simulink model "Nadir_Pointing"  (R2023b)
settings: Solver=VariableStepAuto  StartTime=0.0  StopTime=10.0  RelTol=1e-3
values from neighbouring files (symbols this model uses):
  a = 7259    [Group_51.m]
  a_sun = 149.60e6    (= 149600000)    [Group_51.m]
  ARW = (((arw*pi/180)/(sqrt(n_t)))^2)*n_t    [Group_51.m]
  Beta_CMG = acos(dot([1;0;0],uv_pyr))    [Group_51.m]
  delta_0_P = SM.delta_g_SM(end,:)    [Group_51.m]
  e = 0.001    [Group_51.m]
  e_sun = 0.0167086    [Group_51.m]
  eps_b = 11.5*pi/180    (= 0.200712863979)    [Group_51.m]
  eps_sun = deg2rad(23.45)    [Group_51.m]
  f0_P = SM.Theta_SM(end,1)    [Group_51.m]
  g_1_0 = -29404.8    [Group_51.m]
  g_1_1 = -1450.9    [Group_51.m]
  Gain_G = eye(3,3)    [Group_51.m]
  h_1_1 = 4653.5    [Group_51.m]
  h_r = [0.5;0.5;0.5;0.5]    [Group_51.m]
  halfrange = pi/40    (= 0.0785398163397)    [Group_51.m]
  i = deg2rad(97.27276)    [Group_51.m]
  I_tot = I+Ip_1_transp+Ip_2_transp    [Group_51.m]
  I_tot_inv = I_tot\eye(3,3)    [Group_51.m]
  IC312_P = [phi312_P;theta312_P;psi312_P]    [Group_51.m]
  jb = [0.1; 0.1;0.1]    [Group_51.m]
  k_cmg = -1    [Group_51.m]
  kdx_P = 2    [Group_51.m]
  kdy_P = 2.365    [Group_51.m]
  kdz_P = 2.1    [Group_51.m]
  kpx_SM = 0.129*0.5    (= 0.0645)    [Group_51.m]
  kpy_P = 1.4*0.5    (= 0.7)    [Group_51.m]
  kpz_P = 1*0.5    (= 0.5)    [Group_51.m]
  Miss_G = [teta_g_x;teta_g_y;teta_g_z]    [Group_51.m]
  n = sqrt(mu/ a^3)    [Group_51.m]
  n_sun = 2*pi/(365.26*24*3600)    (= 1.99096676796e-07)    [Group_51.m]
  n_t = samp_t    (= 1)    [Group_51.m]
  OM = deg2rad(90)    [Group_51.m]
  Re = astroConstants(23)    [Group_51.m]
  RRW = (((rrw*pi/180)/(sqrt(n_t)))^2)*n_t    [Group_51.m]
  samp_t = 1/samp_freq    (= 1)    [Group_51.m]
  t_sun_P = tf_D+tf_SM    (= 550)    [Group_51.m]
  w = deg2rad(0)    [Group_51.m]
  w0_P = [wx_P;wy_P;wz_P]    [Group_51.m]
  we = we/3600    (= 7.29159776389e-06)    [Group_51.m]
undefined symbols (not defined in the file or in its folder): DiscIntNeverNeededParam
libraries: matrix_library x15, vrlib x11, simulink x6, hdlsllib x2, dspswit3 x1
(part 2 of 2)

== system Nadir_Pointing/Kinematics/Subsystem/Subsystem4 ==
  angles313 : Inport
  Enable : EnablePort
  Subsystem1 : Subsystem
  Subsystem12 : Subsystem
  angles312 : Outport
  wires:
  Subsystem12/1(Out1) -> Subsystem1/1(matrix313)  "matrix313"
  Subsystem1/1(angles312) -> angles312/1  "angles312"
  angles313/1 -> Subsystem12/1(angles313)

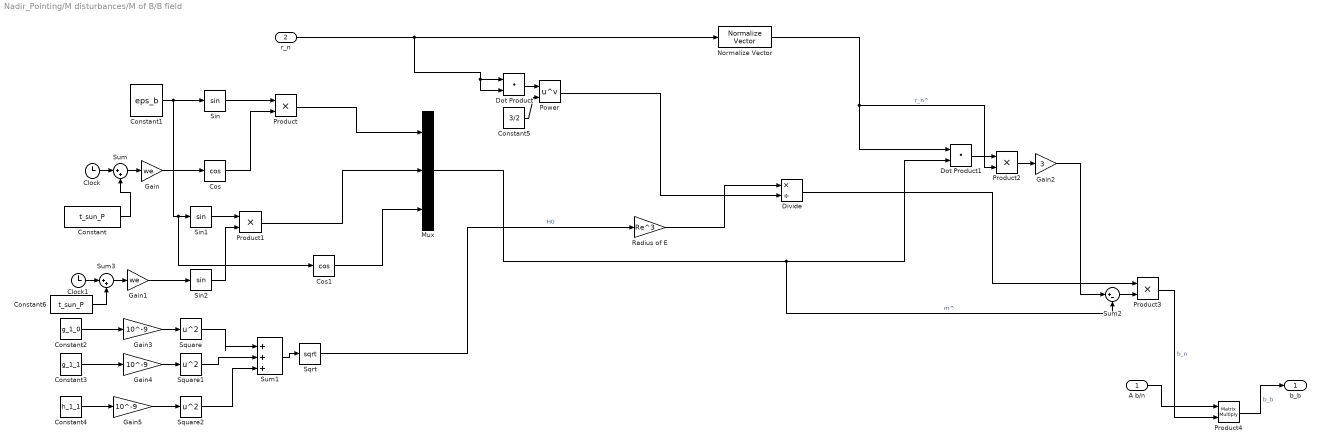
== system Nadir_Pointing/M disturbances/M of B/B field  ==
  A b/n : Inport
  r_n : Inport  Port=2
  Clock : Clock
  Clock1 : Clock
  Constant : Constant  Value=t_sun_P
  Constant1 : Constant  Value=eps_b
  Constant2 : Constant  Value=g_1_0
  Constant3 : Constant  Value=g_1_1
  Constant4 : Constant  Value=h_1_1
  Constant5 : Constant  Value=3/2
  Constant6 : Constant  Value=t_sun_P
  Cos : Trigonometry  Operator=cos
  Cos1 : Trigonometry  Operator=cos
  Divide : Product  Inputs=*/
  Dot Product : DotProduct  OutDataTypeStr=Inherit: Inherit via internal rule
  Dot Product1 : DotProduct  OutDataTypeStr=Inherit: Inherit via internal rule
  Gain : Gain  Gain=we
  Gain1 : Gain  Gain=we
  Gain2 : Gain  Gain=3
  Gain3 : Gain  Gain=10^-9
  Gain4 : Gain  Gain=10^-9
  Gain5 : Gain  Gain=10^-9
  Mux : Mux  Inputs=3
  Normalize Vector : vrlib/Utilities/Normalize Vector  maxzero=0
  Power : Math  Operator=pow
  Product{,1..3} (4 alike) : Product
  Product4 : Product  Multiplication=Matrix(*)
  Radius of E : Gain  Gain=Re^3
  Sin : Trigonometry
  Sin1 : Trigonometry
  Sin2 : Trigonometry
  Sqrt : Sqrt
  Square : Math  Operator=square
  Square1 : Math  Operator=square
  Square2 : Math  Operator=square
  Sum : Sum  Inputs=|++
  Sum1 : Sum  Inputs=|+++
  Sum2 : Sum  Inputs=|+-
  Sum3 : Sum  Inputs=|++
  b_b : Outport
  wires:
  A b/n/1 -> Product4/1
  Product2/1 -> Gain2/1
  Constant5/1 -> Power/2
  Radius of E/1 -> Divide/1
  Normalize Vector/1 -> Product2/2, Dot Product1/1  "r_n^"
  Gain/1 -> Cos/1
  Sum2/1 -> Product3/2
  Sin1/1 -> Product1/1
  Product1/1 -> Mux/2
  Sqrt/1 -> Radius of E/1  "H0"
  Gain1/1 -> Sin2/1
  Sin2/1 -> Product1/2
  Sin/1 -> Product/1
  Product4/1 -> b_b/1  "b_b"
  Cos/1 -> Product/2
  Square2/1 -> Sum1/3
  Constant1/1 -> Cos1/1, Sin1/1, Sin/1
  Cos1/1 -> Mux/3
  Dot Product/1 -> Power/1
  Product3/1 -> Product4/2  "b_n"
  Divide/1 -> Product3/1
  Product/1 -> Mux/1
  Power/1 -> Divide/2
  Sum1/1 -> Sqrt/1
  Dot Product1/1 -> Product2/1
  r_n/1 -> Normalize Vector/1, Dot Product/2, Dot Product/1
  Square1/1 -> Sum1/2
  Square/1 -> Sum1/1
  Mux/1 -> Sum2/2, Dot Product1/2  "m^"
  Gain2/1 -> Sum2/1
  Constant2/1 -> Gain3/1
  Gain3/1 -> Square/1
  Gain4/1 -> Square1/1
  Constant3/1 -> Gain4/1
  Constant4/1 -> Gain5/1
  Gain5/1 -> Square2/1
  Clock/1 -> Sum/1
  Sum/1 -> Gain/1
  Clock1/1 -> Sum3/1
  Sum3/1 -> Gain1/1
  Constant/1 -> Sum/2
  Constant6/1 -> Sum3/2

== system Nadir_Pointing/M disturbances/M of G G/D.C. of R  ==
  Ab/l : Inport
  Product : Product  Multiplication=Matrix(*)
  Yaw Axis : Constant  Value=[1; 0; 0]
  c : Outport
  wires:
  Product/1 -> c/1  "c"
  Ab/l/1 -> Product/1
  Yaw Axis/1 -> Product/2

== system Nadir_Pointing/Sensors/Gyroscopic Sensor/Skew ==
  Theta : Inport
  Constant1 : Constant  Value=[1;0;0]
  Constant2 : Constant  Value=[0;1;0]
  Constant3 : Constant  Value=[0;0;1]
  Cross Product : matrix_library/Cross Product
  Cross Product1 : matrix_library/Cross Product
  Cross Product2 : matrix_library/Cross Product
  Matrix Concatenate : Concatenate  NumInputs=3  Mode=Multidimensional array  ConcatenateDimension=2
  Skew_Theta : Outport
  wires:
  Cross Product/1 -> Matrix Concatenate/1
  Constant3/1 -> Cross Product2/2
  Constant1/1 -> Cross Product/2
  Cross Product1/1 -> Matrix Concatenate/2
  Matrix Concatenate/1 -> Skew_Theta/1
  Theta/1 -> Cross Product1/1, Cross Product2/1, Cross Product/1
  Cross Product2/1 -> Matrix Concatenate/3
  Constant2/1 -> Cross Product1/2

== system Nadir_Pointing/Control/Target Model/Subsystem1/2 A1 rot ==
  ang : Inport
  Constant1 : Constant  Value=[1 0 0; 0 0 0; 0 0 0]
  Constant2 : Constant  Value=[0 0 0; 0 1 0; 0 0 1]
  Constant3 : Constant  Value=[0 0 0; 0 0 1; 0 -1 0]
  Cos : Trigonometry  Operator=cos
  Product : Product
  Product1 : Product
  Sin : Trigonometry
  Sum : Sum  Inputs=|+||+||+
  A21 : Outport
  wires:
  ang/1 -> Sin/1, Cos/1
  Constant3/1 -> Product1/2
  Product1/1 -> Sum/3
  Product/1 -> Sum/2
  Constant1/1 -> Sum/1
  Sin/1 -> Product1/1
  Constant2/1 -> Product/2
  Cos/1 -> Product/1
  Sum/1 -> A21/1

== system Nadir_Pointing/Control/Target Model/Subsystem1/2 A3 rot ==
  ang : Inport
  Constant1 : Constant  Value=[0 0 0; 0 0 0; 0 0 1]
  Constant2 : Constant  Value=[1 0 0; 0 1 0; 0 0 0]
  Constant3 : Constant  Value=[0 1 0; -1 0 0; 0 0 0]
  Cos : Trigonometry  Operator=cos
  Product : Product
  Product1 : Product
  Sin : Trigonometry
  Sum : Sum  Inputs=|+||+||+
  A23 : Outport
  wires:
  Constant2/1 -> Product/2
  Sum/1 -> A23/1
  ang/1 -> Sin/1, Cos/1
  Product/1 -> Sum/2
  Cos/1 -> Product/1
  Sin/1 -> Product1/1
  Constant3/1 -> Product1/2
  Constant1/1 -> Sum/1
  Product1/1 -> Sum/3

== system Nadir_Pointing/Control/Target Model/Subsystem1/2 A3 rot2 ==
  ang : Inport
  Constant1 : Constant  Value=[0 0 0; 0 0 0; 0 0 1]
  Constant2 : Constant  Value=[1 0 0; 0 1 0; 0 0 0]
  Constant3 : Constant  Value=[0 1 0; -1 0 0; 0 0 0]
  Cos : Trigonometry  Operator=cos
  Product : Product
  Product1 : Product
  Sin : Trigonometry
  Sum : Sum  Inputs=|+||+||+
  A233 : Outport
  wires:
  Constant2/1 -> Product/2
  Sum/1 -> A233/1
  ang/1 -> Sin/1, Cos/1
  Product/1 -> Sum/2
  Cos/1 -> Product/1
  Sin/1 -> Product1/1
  Constant3/1 -> Product1/2
  Constant1/1 -> Sum/1
  Product1/1 -> Sum/3

== system Nadir_Pointing/Environment/A l//n for elliptical orbit/Subsystem1/2 A1 rot ==
  ang : Inport
  Constant1 : Constant  Value=[1 0 0; 0 0 0; 0 0 0]
  Constant2 : Constant  Value=[0 0 0; 0 1 0; 0 0 1]
  Constant3 : Constant  Value=[0 0 0; 0 0 1; 0 -1 0]
  Cos : Trigonometry  Operator=cos
  Product : Product
  Product1 : Product
  Sin : Trigonometry
  Sum : Sum  Inputs=|+||+||+
  A21 : Outport
  wires:
  ang/1 -> Sin/1, Cos/1
  Constant3/1 -> Product1/2
  Product1/1 -> Sum/3
  Product/1 -> Sum/2
  Constant1/1 -> Sum/1
  Sin/1 -> Product1/1
  Constant2/1 -> Product/2
  Cos/1 -> Product/1
  Sum/1 -> A21/1

== system Nadir_Pointing/Environment/A l//n for elliptical orbit/Subsystem1/2 A3 rot ==
  ang : Inport
  Constant1 : Constant  Value=[0 0 0; 0 0 0; 0 0 1]
  Constant2 : Constant  Value=[1 0 0; 0 1 0; 0 0 0]
  Constant3 : Constant  Value=[0 1 0; -1 0 0; 0 0 0]
  Cos : Trigonometry  Operator=cos
  Product : Product
  Product1 : Product
  Sin : Trigonometry
  Sum : Sum  Inputs=|+||+||+
  A23 : Outport
  wires:
  Constant2/1 -> Product/2
  Sum/1 -> A23/1
  ang/1 -> Sin/1, Cos/1
  Product/1 -> Sum/2
  Cos/1 -> Product/1
  Sin/1 -> Product1/1
  Constant3/1 -> Product1/2
  Constant1/1 -> Sum/1
  Product1/1 -> Sum/3

== system Nadir_Pointing/Environment/A l//n for elliptical orbit/Subsystem1/2 A3 rot2 ==
  ang : Inport
  Constant1 : Constant  Value=[0 0 0; 0 0 0; 0 0 1]
  Constant2 : Constant  Value=[1 0 0; 0 1 0; 0 0 0]
  Constant3 : Constant  Value=[0 1 0; -1 0 0; 0 0 0]
  Cos : Trigonometry  Operator=cos
  Product : Product
  Product1 : Product
  Sin : Trigonometry
  Sum : Sum  Inputs=|+||+||+
  A233 : Outport
  wires:
  Constant2/1 -> Product/2
  Sum/1 -> A233/1
  ang/1 -> Sin/1, Cos/1
  Product/1 -> Sum/2
  Cos/1 -> Product/1
  Sin/1 -> Product1/1
  Constant3/1 -> Product1/2
  Constant1/1 -> Sum/1
  Product1/1 -> Sum/3

== system Nadir_Pointing/Environment/Kep 2bp/Subsystem/2 A1 rot ==
  theta2 : Inport
  Constant1 : Constant  Value=[1 0 0; 0 0 0; 0 0 0]
  Constant2 : Constant  Value=[0 0 0; 0 1 0; 0 0 1]
  Constant3 : Constant  Value=[0 0 0; 0 0 1; 0 -1 0]
  Cos : Trigonometry  Operator=cos
  Product : Product
  Product1 : Product
  Sin : Trigonometry
  Sum : Sum  Inputs=|+||+||+
  A21 : Outport
  wires:
  theta2/1 -> Sin/1, Cos/1
  Constant3/1 -> Product1/2
  Product1/1 -> Sum/3
  Product/1 -> Sum/2
  Constant1/1 -> Sum/1
  Sin/1 -> Product1/1
  Constant2/1 -> Product/2
  Cos/1 -> Product/1
  Sum/1 -> A21/1

== system Nadir_Pointing/Environment/Kep 2bp/Subsystem/2 A3 rot ==
  angolo : Inport
  Constant1 : Constant  Value=[0 0 0; 0 0 0; 0 0 1]
  Constant2 : Constant  Value=[1 0 0; 0 1 0; 0 0 0]
  Constant3 : Constant  Value=[0 1 0; -1 0 0; 0 0 0]
  Cos : Trigonometry  Operator=cos
  Product : Product
  Product1 : Product
  Sin : Trigonometry
  Sum : Sum  Inputs=|+||+||+
  A23 : Outport
  wires:
  Constant2/1 -> Product/2
  Sum/1 -> A23/1
  angolo/1 -> Sin/1, Cos/1
  Product/1 -> Sum/2
  Cos/1 -> Product/1
  Sin/1 -> Product1/1
  Constant3/1 -> Product1/2
  Constant1/1 -> Sum/1
  Product1/1 -> Sum/3

== system Nadir_Pointing/Environment/Kep 2bp/Subsystem/2 A3 rot2 ==
  angolo : Inport
  Constant1 : Constant  Value=[0 0 0; 0 0 0; 0 0 1]
  Constant2 : Constant  Value=[1 0 0; 0 1 0; 0 0 0]
  Constant3 : Constant  Value=[0 1 0; -1 0 0; 0 0 0]
  Cos : Trigonometry  Operator=cos
  Product : Product
  Product1 : Product
  Sin : Trigonometry
  Sum : Sum  Inputs=|+||+||+
  A233 : Outport
  wires:
  Constant2/1 -> Product/2
  Sum/1 -> A233/1
  angolo/1 -> Sin/1, Cos/1
  Product/1 -> Sum/2
  Cos/1 -> Product/1
  Sin/1 -> Product1/1
  Constant3/1 -> Product1/2
  Constant1/1 -> Sum/1
  Product1/1 -> Sum/3

== system Nadir_Pointing/Kinematics/Euler Angles/Kinematics 312/Subsystem1 ==
  wx : Inport
  theta : Inport  Port=2
  wz : Inport  Port=3
  psi : Inport  Port=4
  Cos : Trigonometry  Operator=cos
  Cos1 : Trigonometry  Operator=cos
  Divide : Product  Inputs=*/
  Product : Product
  Product1 : Product
  Sin : Trigonometry
  Sum : Sum  Inputs=|+-
  Out1 : Outport
  wires:
  psi/1 -> Cos/1, Sin/1
  theta/1 -> Cos1/1
  Product1/1 -> Sum/2
  Sum/1 -> Divide/1
  Product/1 -> Sum/1
  Sin/1 -> Product1/1
  Cos1/1 -> Divide/2
  Cos/1 -> Product/2
  wx/1 -> Product1/2
  wz/1 -> Product/1
  Divide/1 -> Out1/1  "phidot"

== system Nadir_Pointing/Kinematics/Euler Angles/Kinematics 312/Subsystem3 ==
  wx : Inport
  wy : Inport  Port=2
  theta : Inport  Port=3
  psi : Inport  Port=4
  wz : Inport  Port=5
  Cos : Trigonometry  Operator=cos
  Cos1 : Trigonometry  Operator=cos
  Divide : Product  Inputs=*/
  Product : Product
  Product1 : Product
  Product2 : Product
  Sin : Trigonometry
  Sin1 : Trigonometry
  Subtract : Sum  Inputs=+-
  Subtract1 : Sum  Inputs=+-
  Out1 : Outport
  wires:
  psi/1 -> Cos/1, Sin/1
  Subtract/1 -> Product2/1
  Sin1/1 -> Divide/1
  Product2/1 -> Subtract1/2
  Sin/1 -> Product1/1
  Cos/1 -> Product/2
  Cos1/1 -> Divide/2
  Subtract1/1 -> Out1/1  "psidot"
  wz/1 -> Product/1
  theta/1 -> Sin1/1, Cos1/1
  Product1/1 -> Subtract/2
  Divide/1 -> Product2/2
  Product/1 -> Subtract/1
  wy/1 -> Subtract1/1
  wx/1 -> Product1/2

== system Nadir_Pointing/Kinematics/Euler Angles/Kinematics 312/Subsystem4 ==
  wx : Inport
  wz : Inport  Port=2
  psi : Inport  Port=3
  Cos : Trigonometry  Operator=cos
  Product : Product
  Product1 : Product
  Sin : Trigonometry
  Sum : Sum  Inputs=|++
  Out1 : Outport
  wires:
  Sum/1 -> Out1/1  "thetadot"
  Sin/1 -> Product1/1
  psi/1 -> Sin/1, Cos/1
  Product/1 -> Sum/1
  Product1/1 -> Sum/2
  wx/1 -> Product/1
  Cos/1 -> Product/2
  wz/1 -> Product1/2

== system Nadir_Pointing/Kinematics/Euler Angles/Kinematics 312/Subsystem5 ==
  psi312 : Inport
  Constant1 : Constant  Value=[0 0 0; 0 1 0; 0 0 0]
  Constant2 : Constant  Value=[0 0 -1; 0 0 0; 1 0 0]
  Constant3 : Constant  Value=[1 0 0; 0 0 0; 0 0 1]
  Cos : Trigonometry  Operator=cos
  Product : Product
  Product1 : Product
  Sin : Trigonometry
  Sum : Sum  Inputs=|+++
  2 : Outport
  wires:
  Sum/1 -> 2/1  "A2psi"
  psi312/1 -> Cos/1, Sin/1  "psi"
  Constant1/1 -> Sum/1
  Product/1 -> Sum/2
  Constant2/1 -> Product/2
  Sin/1 -> Product/1
  Cos/1 -> Product1/1
  Constant3/1 -> Product1/2
  Product1/1 -> Sum/3

== system Nadir_Pointing/Kinematics/Euler Angles/Kinematics 312/Subsystem7 ==
  theta312 : Inport
  Constant1 : Constant  Value=[1 0 0; 0 0 0; 0 0 0]
  Constant2 : Constant  Value=[0 0 0; 0 0 1; 0 -1 0]
  Constant3 : Constant  Value=[0 0 0; 0 1 0; 0 0 1]
  Cos : Trigonometry  Operator=cos
  Product : Product
  Product1 : Product
  Sin : Trigonometry
  Sum : Sum  Inputs=|+++
  1 : Outport
  wires:
  theta312/1 -> Cos/1, Sin/1
  Sum/1 -> 1/1  "A1theta"
  Constant1/1 -> Sum/1
  Sin/1 -> Product/1
  Constant2/1 -> Product/2
  Product/1 -> Sum/2
  Cos/1 -> Product1/1
  Constant3/1 -> Product1/2
  Product1/1 -> Sum/3

== system Nadir_Pointing/Kinematics/Euler Angles/Kinematics 312/Subsystem9 ==
  phi312 : Inport
  Constant1 : Constant  Value=[0 0 0; 0 0 0; 0 0 1]
  Constant2 : Constant  Value=[0 1 0; -1 0 0; 0 0 0]
  Constant3 : Constant  Value=[1 0 0; 0 1 0; 0 0 0]
  Cos : Trigonometry  Operator=cos
  Product : Product
  Product1 : Product
  Sin : Trigonometry
  Sum : Sum  Inputs=|+++
  3 : Outport
  wires:
  phi312/1 -> Cos/1, Sin/1
  Constant1/1 -> Sum/1
  Sum/1 -> 3/1  "A3phi"
  Sin/1 -> Product/1
  Constant2/1 -> Product/2
  Product/1 -> Sum/2
  Cos/1 -> Product1/1
  Constant3/1 -> Product1/2
  Product1/1 -> Sum/3

== system Nadir_Pointing/Kinematics/Euler Angles/Kinematics 313/Subsystem1 ==
  wx : Inport
  wy : Inport  Port=2
  psi : Inport  Port=3
  Cos : Trigonometry  Operator=cos
  Product : Product
  Product1 : Product
  Sin : Trigonometry
  Subtract : Sum  Inputs=-+
  thetadot : Outport
  wires:
  Product/1 -> Subtract/1
  Product1/1 -> Subtract/2
  psi/1 -> Sin/1, Cos/1
  wy/1 -> Product/1
  wx/1 -> Product1/2
  Cos/1 -> Product1/1
  Subtract/1 -> thetadot/1  "thetadot"
  Sin/1 -> Product/2

== system Nadir_Pointing/Kinematics/Euler Angles/Kinematics 313/Subsystem2 ==
  wx : Inport
  wy : Inport  Port=2
  theta : Inport  Port=3
  psi : Inport  Port=4
  Cos : Trigonometry  Operator=cos
  Cos1 : Trigonometry
  Divide : Product  Inputs=*/
  Product : Product
  Product1 : Product
  Sin : Trigonometry
  Sum : Sum  Inputs=|++
  phidot : Outport
  wires:
  psi/1 -> Cos/1, Sin/1
  Cos/1 -> Product/1
  Sum/1 -> Divide/1
  Cos1/1 -> Divide/2
  Product/1 -> Sum/2
  Product1/1 -> Sum/1
  Sin/1 -> Product1/1
  wx/1 -> Product1/2
  wy/1 -> Product/2
  Divide/1 -> phidot/1  "phidot"
  theta/1 -> Cos1/1

== system Nadir_Pointing/Kinematics/Euler Angles/Kinematics 313/Subsystem3 ==
  wx : Inport
  wy : Inport  Port=2
  theta : Inport  Port=3
  wz : Inport  Port=4
  psi : Inport  Port=5
  Cos : Trigonometry  Operator=cos
  Cos1 : Trigonometry
  Cos2 : Trigonometry  Operator=cos
  Cos3 : Trigonometry
  Divide : Product  Inputs=*/
  Product : Product
  Product1 : Product
  Product2 : Product
  Sum : Sum  Inputs=|++
  Sum1 : Sum  Inputs=+-
  psidot : Outport
  wires:
  theta/1 -> Cos3/1, Cos2/1
  Product2/1 -> Sum1/2
  Cos/1 -> Product1/1
  Product/1 -> Sum/1
  Cos2/1 -> Divide/1
  psi/1 -> Cos/1, Cos1/1
  Cos3/1 -> Divide/2
  Divide/1 -> Product2/2
  Sum/1 -> Product2/1
  wy/1 -> Product1/2
  Product1/1 -> Sum/2
  Sum1/1 -> psidot/1  "psidot"
  wz/1 -> Sum1/1
  Cos1/1 -> Product/2
  wx/1 -> Product/1

== system Nadir_Pointing/Kinematics/Euler Angles/Kinematics 313/Subsystem4 ==
  theta : Inport
  Constant1 : Constant  Value=[1 0 0; 0 0 0; 0 0 0]
  Constant2 : Constant  Value=[0 0 0; 0 0 1; 0 -1 0]
  Constant3 : Constant  Value=[0 0 0; 0 1 0; 0 0 1]
  Cos : Trigonometry  Operator=cos
  Product : Product
  Product1 : Product
  Sin : Trigonometry
  Sum : Sum  Inputs=|+++
  1 : Outport
  wires:
  theta/1 -> Cos/1, Sin/1
  Sum/1 -> 1/1  "A1theta"
  Constant1/1 -> Sum/1
  Sin/1 -> Product/1
  Constant2/1 -> Product/2
  Product/1 -> Sum/2
  Cos/1 -> Product1/1
  Constant3/1 -> Product1/2
  Product1/1 -> Sum/3

== system Nadir_Pointing/Kinematics/Euler Angles/Kinematics 313/Subsystem5 ==
  psi : Inport
  Constant1 : Constant  Value=[0 0 0; 0 0 0; 0 0 1]
  Constant2 : Constant  Value=[0 1 0; -1 0 0; 0 0 0]
  Constant3 : Constant  Value=[1 0 0; 0 1 0; 0 0 0]
  Cos : Trigonometry  Operator=cos
  Product : Product
  Product1 : Product
  Sin : Trigonometry
  Sum : Sum  Inputs=|+++
  3 : Outport
  wires:
  Sum/1 -> 3/1  "A3psi"
  psi/1 -> Sin/1, Cos/1  "psi"
  Product1/1 -> Sum/3
  Constant3/1 -> Product1/2
  Sin/1 -> Product/1
  Constant2/1 -> Product/2
  Cos/1 -> Product1/1
  Product/1 -> Sum/2
  Constant1/1 -> Sum/1

== system Nadir_Pointing/Kinematics/Euler Angles/Kinematics 313/Subsystem6 ==
  phi : Inport
  Constant1 : Constant  Value=[0 0 0; 0 0 0; 0 0 1]
  Constant2 : Constant  Value=[0 1 0; -1 0 0; 0 0 0]
  Constant3 : Constant  Value=[1 0 0; 0 1 0; 0 0 0]
  Cos : Trigonometry  Operator=cos
  Product : Product
  Product1 : Product
  Sin : Trigonometry
  Sum : Sum  Inputs=|+++
  3 : Outport
  wires:
  phi/1 -> Cos/1, Sin/1
  Constant1/1 -> Sum/1
  Sum/1 -> 3/1  "A3phi"
  Sin/1 -> Product/1
  Constant2/1 -> Product/2
  Product/1 -> Sum/2
  Cos/1 -> Product1/1
  Constant3/1 -> Product1/2
  Product1/1 -> Sum/3

== system Nadir_Pointing/Kinematics/Euler Angles/Subsystem3/Subsystem10 ==
  In1 : Inport
  Atan2 : Trigonometry  Operator=atan2
  Atan5 : Trigonometry  Operator=atan2
  Atan6 : Trigonometry  Operator=atan2
  Divide1 : Product  Inputs=*/
  Gain3 : Gain  Gain=-1
  Mux2 : Mux  Inputs=3
  Selector12 : Selector  NumberOfDimensions=2  InputPortWidth=3  IndexOptions=Index vector (dialog),Index vector (dialog)  Indices=3,1  OutputSizes=1,1
  Selector13 : Selector  NumberOfDimensions=2  InputPortWidth=3  IndexOptions=Index vector (dialog),Index vector (dialog)  Indices=3,2  OutputSizes=1,1
  Selector14 : Selector  NumberOfDimensions=2  InputPortWidth=3  IndexOptions=Index vector (dialog),Index vector (dialog)  Indices=1,3  OutputSizes=1,1
  Selector15 : Selector  NumberOfDimensions=2  InputPortWidth=3  IndexOptions=Index vector (dialog),Index vector (dialog)  Indices=2,3  OutputSizes=1,1
  Selector5 : Selector  NumberOfDimensions=2  InputPortWidth=3  IndexOptions=Index vector (dialog),Index vector (dialog)  Indices=3,3  OutputSizes=1,1
  Square Root1 : Sqrt
  Square4 : Math  Operator=square
  Square5 : Math  Operator=square
  Sum2 : Sum  Inputs=|++
  Tan2 : Trigonometry  Operator=atan
  angles313 : Outport
  wires:
  Square Root1/1 -> Atan6/1
  In1/1 -> Selector15/1, Selector14/1, Selector13/1, Selector5/1, Selector12/1  "matrix312"
  Atan5/1 -> Mux2/3  "psicheck"
  Selector13/1 -> Atan2/2, Divide1/2, Square5/1  "a32"
  Selector14/1 -> Atan5/1  "a13"
  Square5/1 -> Sum2/2
  Selector5/1 -> Atan6/2  "a33"
  Gain3/1 -> Mux2/1  "phicheck"
  Selector12/1 -> Atan2/1, Divide1/1, Square4/1  "a31"
  Selector15/1 -> Atan5/2  "a23"
  Atan6/1 -> Mux2/2  "thetacheck"
  Sum2/1 -> Square Root1/1
  Square4/1 -> Sum2/1
  Mux2/1 -> angles313/1  "angles313"
  Divide1/1 -> Tan2/1
  Atan2/1 -> Gain3/1

== system Nadir_Pointing/Kinematics/Euler Angles/Subsystem3/Subsystem12 ==
  angles313 : Inport
  Demux5 : Demux  Outputs=3
  Matrix Multiply1 : Product  Inputs=3  Multiplication=Matrix(*)
  Subsystem4 : Subsystem
  Subsystem5 : Subsystem
  Subsystem6 : Subsystem
  Out1 : Outport
  wires:
  Demux5/1 -> Subsystem6/1(phi)
  Subsystem4/1(1) -> Matrix Multiply1/2
  Subsystem6/1(3) -> Matrix Multiply1/3
  angles313/1 -> Demux5/1
  Subsystem5/1(3) -> Matrix Multiply1/1
  Demux5/3 -> Subsystem5/1(psi)
  Demux5/2 -> Subsystem4/1(theta)
  Matrix Multiply1/1 -> Out1/1  "matrix313"

== system Nadir_Pointing/Kinematics/Euler Angles/Subsystem3/Subsystem4 ==
  matrix313 : Inport
  Atan1 : Trigonometry  Operator=atan2
  Atan2 : Trigonometry  Operator=atan2
  Atan3 : Trigonometry  Operator=atan2
  Divide : Product  Inputs=*/
  Gain : Gain  Gain=-1
  Mux : Mux  Inputs=3
  Selector : Selector  NumberOfDimensions=2  InputPortWidth=3  IndexOptions=Index vector (dialog),Index vector (dialog)  Indices=3,3  OutputSizes=1,1
  Selector1 : Selector  NumberOfDimensions=2  InputPortWidth=3  IndexOptions=Index vector (dialog),Index vector (dialog)  Indices=3,1  OutputSizes=1,1
  Selector2 : Selector  NumberOfDimensions=2  InputPortWidth=3  IndexOptions=Index vector (dialog),Index vector (dialog)  Indices=3,2  OutputSizes=1,1
  Selector3 : Selector  NumberOfDimensions=2  InputPortWidth=3  IndexOptions=Index vector (dialog),Index vector (dialog)  Indices=1,3  OutputSizes=1,1
  Selector4 : Selector  NumberOfDimensions=2  InputPortWidth=3  IndexOptions=Index vector (dialog),Index vector (dialog)  Indices=2,3  OutputSizes=1,1
  Square : Math  Operator=square
  Square Root : Sqrt
  Square1 : Math  Operator=square
  Sum : Sum  Inputs=|++
  Tan : Trigonometry  Operator=atan
  angles313 : Outport
  wires:
  Atan1/1 -> Mux/3  "psicheck"
  Selector/1 -> Atan2/2  "a33"
  Square Root/1 -> Atan2/1
  Square1/1 -> Sum/2
  Square/1 -> Sum/1
  Selector4/1 -> Atan1/2  "a23"
  Sum/1 -> Square Root/1
  matrix313/1 -> Selector/1, Selector2/1, Selector3/1, Selector4/1, Selector1/1
  Gain/1 -> Mux/1  "phicheck"
  Selector3/1 -> Atan1/1  "a13"
  Selector2/1 -> Atan3/2, Divide/2, Square1/1  "a32"
  Divide/1 -> Tan/1
  Selector1/1 -> Atan3/1, Divide/1, Square/1  "a31"
  Atan2/1 -> Mux/2  "thetacheck"
  Mux/1 -> angles313/1  "angles313"
  Atan3/1 -> Gain/1

== system Nadir_Pointing/Kinematics/Euler Angles/Subsystem3/Subsystem6 ==
  In1 : Inport
  Demux : Demux  Outputs=3
  Matrix Multiply : Product  Inputs=3  Multiplication=Matrix(*)
  Subsystem7 : Subsystem
  Subsystem8 : Subsystem
  Subsystem9 : Subsystem
  Out1 : Outport
  wires:
  Subsystem7/1(2) -> Matrix Multiply/1
  Demux/1 -> Subsystem9/1(phi312)
  Demux/3 -> Subsystem7/1(psi312)
  Demux/2 -> Subsystem8/1(theta312)
  Subsystem8/1(1) -> Matrix Multiply/2
  Subsystem9/1(3) -> Matrix Multiply/3
  In1/1 -> Demux/1
  Matrix Multiply/1 -> Out1/1  "matrix312"

== system Nadir_Pointing/Kinematics/Euler Angles/Subsystem4/Subsystem1 ==
  matrix313 : Inport
  Atan3 : Trigonometry  Operator=atan2
  Atan4 : Trigonometry  Operator=atan2
  Display2 : Display
  Gain1 : Gain  Gain=-1
  Gain2 : Gain  Gain=-1
  Mux1 : Mux  Inputs=3
  Selector10 : Selector  NumberOfDimensions=2  InputPortWidth=3  IndexOptions=Index vector (dialog),Index vector (dialog)  Indices=1,3  OutputSizes=1,1
  Selector11 : Selector  NumberOfDimensions=2  InputPortWidth=3  IndexOptions=Index vector (dialog),Index vector (dialog)  Indices=3,3  OutputSizes=1,1
  Selector6 : Selector  NumberOfDimensions=2  InputPortWidth=3  IndexOptions=Index vector (dialog),Index vector (dialog)  Indices=3,3  OutputSizes=1,1
  Selector7 : Selector  NumberOfDimensions=2  InputPortWidth=3  IndexOptions=Index vector (dialog),Index vector (dialog)  Indices=2,3  OutputSizes=1,1
  Selector8 : Selector  NumberOfDimensions=2  InputPortWidth=3  IndexOptions=Index vector (dialog),Index vector (dialog)  Indices=2,1  OutputSizes=1,1
  Selector9 : Selector  NumberOfDimensions=2  InputPortWidth=3  IndexOptions=Index vector (dialog),Index vector (dialog)  Indices=2,2  OutputSizes=1,1
  Sqrt : Sqrt
  Square2 : Math  Operator=square
  Square3 : Math  Operator=square
  Sum1 : Sum  Inputs=|++
  Tan1 : Trigonometry  Operator=atan2
  angles312 : Outport
  wires:
  Selector9/1 -> Square3/1, Tan1/2  "a22"
  Sqrt/1 -> Atan3/2
  matrix313/1 -> Selector7/1, Selector8/1, Selector9/1, Selector11/1, Selector10/1, Selector6/1
  Selector8/1 -> Tan1/1, Square2/1  "a21"
  Selector10/1 -> Atan4/1  "a13"
  Gain2/1 -> Mux1/3  "psicheck"
  Square2/1 -> Sum1/1
  Sum1/1 -> Sqrt/1
  Selector11/1 -> Atan4/2  "a33"
  Selector6/1 -> Display2/1
  Square3/1 -> Sum1/2
  Selector7/1 -> Atan3/1  "a23"
  Atan4/1 -> Gain2/1
  Tan1/1 -> Gain1/1
  Atan3/1 -> Mux1/2  "thetacheck"
  Gain1/1 -> Mux1/1  "phicheck"
  Mux1/1 -> angles312/1  "angles312"

== system Nadir_Pointing/Kinematics/Euler Angles/Subsystem4/Subsystem12 ==
  angles313 : Inport
  Demux5 : Demux  Outputs=3
  Matrix Multiply1 : Product  Inputs=3  Multiplication=Matrix(*)
  Subsystem4 : Subsystem
  Subsystem5 : Subsystem
  Subsystem6 : Subsystem
  Out1 : Outport
  wires:
  Demux5/1 -> Subsystem6/1(phi)
  Subsystem4/1(1) -> Matrix Multiply1/2
  Subsystem6/1(3) -> Matrix Multiply1/3
  angles313/1 -> Demux5/1
  Subsystem5/1(3) -> Matrix Multiply1/1
  Demux5/3 -> Subsystem5/1(psi)
  Demux5/2 -> Subsystem4/1(theta)
  Matrix Multiply1/1 -> Out1/1  "matrix313"

== system Nadir_Pointing/Kinematics/Subsystem/Subsystem4/Subsystem1 ==
  matrix313 : Inport
  Atan3 : Trigonometry  Operator=atan2
  Atan4 : Trigonometry  Operator=atan2
  Display2 : Display
  Gain1 : Gain  Gain=-1
  Gain2 : Gain  Gain=-1
  Mux1 : Mux  Inputs=3
  Selector10 : Selector  NumberOfDimensions=2  InputPortWidth=3  IndexOptions=Index vector (dialog),Index vector (dialog)  Indices=1,3  OutputSizes=1,1
  Selector11 : Selector  NumberOfDimensions=2  InputPortWidth=3  IndexOptions=Index vector (dialog),Index vector (dialog)  Indices=3,3  OutputSizes=1,1
  Selector6 : Selector  NumberOfDimensions=2  InputPortWidth=3  IndexOptions=Index vector (dialog),Index vector (dialog)  Indices=3,3  OutputSizes=1,1
  Selector7 : Selector  NumberOfDimensions=2  InputPortWidth=3  IndexOptions=Index vector (dialog),Index vector (dialog)  Indices=2,3  OutputSizes=1,1
  Selector8 : Selector  NumberOfDimensions=2  InputPortWidth=3  IndexOptions=Index vector (dialog),Index vector (dialog)  Indices=2,1  OutputSizes=1,1
  Selector9 : Selector  NumberOfDimensions=2  InputPortWidth=3  IndexOptions=Index vector (dialog),Index vector (dialog)  Indices=2,2  OutputSizes=1,1
  Sqrt : Sqrt
  Square2 : Math  Operator=square
  Square3 : Math  Operator=square
  Sum1 : Sum  Inputs=|++
  Tan1 : Trigonometry  Operator=atan2
  angles312 : Outport
  wires:
  Selector9/1 -> Square3/1, Tan1/2  "a22"
  Sqrt/1 -> Atan3/2
  matrix313/1 -> Selector7/1, Selector8/1, Selector9/1, Selector11/1, Selector10/1, Selector6/1
  Selector8/1 -> Tan1/1, Square2/1  "a21"
  Selector10/1 -> Atan4/1  "a13"
  Gain2/1 -> Mux1/3  "psicheck"
  Square2/1 -> Sum1/1
  Sum1/1 -> Sqrt/1
  Selector11/1 -> Atan4/2  "a33"
  Selector6/1 -> Display2/1
  Square3/1 -> Sum1/2
  Selector7/1 -> Atan3/1  "a23"
  Atan4/1 -> Gain2/1
  Tan1/1 -> Gain1/1
  Atan3/1 -> Mux1/2  "thetacheck"
  Gain1/1 -> Mux1/1  "phicheck"
  Mux1/1 -> angles312/1  "angles312"

== system Nadir_Pointing/Kinematics/Subsystem/Subsystem4/Subsystem12 ==
  angles313 : Inport
  Demux5 : Demux  Outputs=3
  Matrix Multiply1 : Product  Inputs=3  Multiplication=Matrix(*)
  Subsystem4 : Subsystem
  Subsystem5 : Subsystem
  Subsystem6 : Subsystem
  Out1 : Outport
  wires:
  Demux5/1 -> Subsystem6/1(phi)
  Subsystem4/1(1) -> Matrix Multiply1/2
  Subsystem6/1(3) -> Matrix Multiply1/3
  angles313/1 -> Demux5/1
  Subsystem5/1(3) -> Matrix Multiply1/1
  Demux5/3 -> Subsystem5/1(psi)
  Demux5/2 -> Subsystem4/1(theta)
  Matrix Multiply1/1 -> Out1/1  "matrix313"

== system Nadir_Pointing/Kinematics/Euler Angles/Subsystem3/Subsystem12/Subsystem4 ==
  theta : Inport
  Constant1 : Constant  Value=[1 0 0; 0 0 0; 0 0 0]
  Constant2 : Constant  Value=[0 0 0; 0 0 1; 0 -1 0]
  Constant3 : Constant  Value=[0 0 0; 0 1 0; 0 0 1]
  Cos : Trigonometry  Operator=cos
  Product : Product
  Product1 : Product
  Sin : Trigonometry
  Sum : Sum  Inputs=|+++
  1 : Outport
  wires:
  theta/1 -> Cos/1, Sin/1
  Sum/1 -> 1/1  "A1theta"
  Constant1/1 -> Sum/1
  Sin/1 -> Product/1
  Constant2/1 -> Product/2
  Product/1 -> Sum/2
  Cos/1 -> Product1/1
  Constant3/1 -> Product1/2
  Product1/1 -> Sum/3

== system Nadir_Pointing/Kinematics/Euler Angles/Subsystem3/Subsystem12/Subsystem5 ==
  psi : Inport
  Constant1 : Constant  Value=[0 0 0; 0 0 0; 0 0 1]
  Constant2 : Constant  Value=[0 1 0; -1 0 0; 0 0 0]
  Constant3 : Constant  Value=[1 0 0; 0 1 0; 0 0 0]
  Cos : Trigonometry  Operator=cos
  Product : Product
  Product1 : Product
  Sin : Trigonometry
  Sum : Sum  Inputs=|+++
  3 : Outport
  wires:
  Sum/1 -> 3/1  "A3psi"
  psi/1 -> Sin/1, Cos/1  "psi"
  Product1/1 -> Sum/3
  Constant3/1 -> Product1/2
  Sin/1 -> Product/1
  Constant2/1 -> Product/2
  Cos/1 -> Product1/1
  Product/1 -> Sum/2
  Constant1/1 -> Sum/1

== system Nadir_Pointing/Kinematics/Euler Angles/Subsystem3/Subsystem12/Subsystem6 ==
  phi : Inport
  Constant1 : Constant  Value=[0 0 0; 0 0 0; 0 0 1]
  Constant2 : Constant  Value=[0 1 0; -1 0 0; 0 0 0]
  Constant3 : Constant  Value=[1 0 0; 0 1 0; 0 0 0]
  Cos : Trigonometry  Operator=cos
  Product : Product
  Product1 : Product
  Sin : Trigonometry
  Sum : Sum  Inputs=|+++
  3 : Outport
  wires:
  phi/1 -> Cos/1, Sin/1
  Constant1/1 -> Sum/1
  Sum/1 -> 3/1  "A3phi"
  Sin/1 -> Product/1
  Constant2/1 -> Product/2
  Product/1 -> Sum/2
  Cos/1 -> Product1/1
  Constant3/1 -> Product1/2
  Product1/1 -> Sum/3

== system Nadir_Pointing/Kinematics/Euler Angles/Subsystem3/Subsystem6/Subsystem7 ==
  psi312 : Inport
  Constant1 : Constant  Value=[0 0 0; 0 1 0; 0 0 0]
  Constant2 : Constant  Value=[0 0 -1; 0 0 0; 1 0 0]
  Constant3 : Constant  Value=[1 0 0; 0 0 0; 0 0 1]
  Cos : Trigonometry  Operator=cos
  Product : Product
  Product1 : Product
  Sin : Trigonometry
  Sum : Sum  Inputs=|+++
  2 : Outport
  wires:
  Sum/1 -> 2/1  "A2psi"
  psi312/1 -> Cos/1, Sin/1  "psi"
  Constant1/1 -> Sum/1
  Product/1 -> Sum/2
  Constant2/1 -> Product/2
  Sin/1 -> Product/1
  Cos/1 -> Product1/1
  Constant3/1 -> Product1/2
  Product1/1 -> Sum/3

== system Nadir_Pointing/Kinematics/Euler Angles/Subsystem3/Subsystem6/Subsystem8 ==
  theta312 : Inport
  Constant1 : Constant  Value=[1 0 0; 0 0 0; 0 0 0]
  Constant2 : Constant  Value=[0 0 0; 0 0 1; 0 -1 0]
  Constant3 : Constant  Value=[0 0 0; 0 1 0; 0 0 1]
  Cos : Trigonometry  Operator=cos
  Product : Product
  Product1 : Product
  Sin : Trigonometry
  Sum : Sum  Inputs=|+++
  1 : Outport
  wires:
  theta312/1 -> Cos/1, Sin/1
  Sum/1 -> 1/1  "A1theta"
  Constant1/1 -> Sum/1
  Sin/1 -> Product/1
  Constant2/1 -> Product/2
  Product/1 -> Sum/2
  Cos/1 -> Product1/1
  Constant3/1 -> Product1/2
  Product1/1 -> Sum/3

== system Nadir_Pointing/Kinematics/Euler Angles/Subsystem3/Subsystem6/Subsystem9 ==
  phi312 : Inport
  Constant1 : Constant  Value=[0 0 0; 0 0 0; 0 0 1]
  Constant2 : Constant  Value=[0 1 0; -1 0 0; 0 0 0]
  Constant3 : Constant  Value=[1 0 0; 0 1 0; 0 0 0]
  Cos : Trigonometry  Operator=cos
  Product : Product
  Product1 : Product
  Sin : Trigonometry
  Sum : Sum  Inputs=|+++
  3 : Outport
  wires:
  phi312/1 -> Cos/1, Sin/1
  Constant1/1 -> Sum/1
  Sum/1 -> 3/1  "A3phi"
  Sin/1 -> Product/1
  Constant2/1 -> Product/2
  Product/1 -> Sum/2
  Cos/1 -> Product1/1
  Constant3/1 -> Product1/2
  Product1/1 -> Sum/3

== system Nadir_Pointing/Kinematics/Euler Angles/Subsystem4/Subsystem12/Subsystem4 ==
  theta : Inport
  Constant1 : Constant  Value=[1 0 0; 0 0 0; 0 0 0]
  Constant2 : Constant  Value=[0 0 0; 0 0 1; 0 -1 0]
  Constant3 : Constant  Value=[0 0 0; 0 1 0; 0 0 1]
  Cos : Trigonometry  Operator=cos
  Product : Product
  Product1 : Product
  Sin : Trigonometry
  Sum : Sum  Inputs=|+++
  1 : Outport
  wires:
  theta/1 -> Cos/1, Sin/1
  Sum/1 -> 1/1  "A1theta"
  Constant1/1 -> Sum/1
  Sin/1 -> Product/1
  Constant2/1 -> Product/2
  Product/1 -> Sum/2
  Cos/1 -> Product1/1
  Constant3/1 -> Product1/2
  Product1/1 -> Sum/3

== system Nadir_Pointing/Kinematics/Euler Angles/Subsystem4/Subsystem12/Subsystem5 ==
  psi : Inport
  Constant1 : Constant  Value=[0 0 0; 0 0 0; 0 0 1]
  Constant2 : Constant  Value=[0 1 0; -1 0 0; 0 0 0]
  Constant3 : Constant  Value=[1 0 0; 0 1 0; 0 0 0]
  Cos : Trigonometry  Operator=cos
  Product : Product
  Product1 : Product
  Sin : Trigonometry
  Sum : Sum  Inputs=|+++
  3 : Outport
  wires:
  Sum/1 -> 3/1  "A3psi"
  psi/1 -> Sin/1, Cos/1  "psi"
  Product1/1 -> Sum/3
  Constant3/1 -> Product1/2
  Sin/1 -> Product/1
  Constant2/1 -> Product/2
  Cos/1 -> Product1/1
  Product/1 -> Sum/2
  Constant1/1 -> Sum/1

== system Nadir_Pointing/Kinematics/Euler Angles/Subsystem4/Subsystem12/Subsystem6 ==
  phi : Inport
  Constant1 : Constant  Value=[0 0 0; 0 0 0; 0 0 1]
  Constant2 : Constant  Value=[0 1 0; -1 0 0; 0 0 0]
  Constant3 : Constant  Value=[1 0 0; 0 1 0; 0 0 0]
  Cos : Trigonometry  Operator=cos
  Product : Product
  Product1 : Product
  Sin : Trigonometry
  Sum : Sum  Inputs=|+++
  3 : Outport
  wires:
  phi/1 -> Cos/1, Sin/1
  Constant1/1 -> Sum/1
  Sum/1 -> 3/1  "A3phi"
  Sin/1 -> Product/1
  Constant2/1 -> Product/2
  Product/1 -> Sum/2
  Cos/1 -> Product1/1
  Constant3/1 -> Product1/2
  Product1/1 -> Sum/3

== system Nadir_Pointing/Kinematics/Subsystem/Subsystem4/Subsystem12/Subsystem4 ==
  theta : Inport
  Constant1 : Constant  Value=[1 0 0; 0 0 0; 0 0 0]
  Constant2 : Constant  Value=[0 0 0; 0 0 1; 0 -1 0]
  Constant3 : Constant  Value=[0 0 0; 0 1 0; 0 0 1]
  Cos : Trigonometry  Operator=cos
  Product : Product
  Product1 : Product
  Sin : Trigonometry
  Sum : Sum  Inputs=|+++
  1 : Outport
  wires:
  theta/1 -> Cos/1, Sin/1
  Sum/1 -> 1/1  "A1theta"
  Constant1/1 -> Sum/1
  Sin/1 -> Product/1
  Constant2/1 -> Product/2
  Product/1 -> Sum/2
  Cos/1 -> Product1/1
  Constant3/1 -> Product1/2
  Product1/1 -> Sum/3

== system Nadir_Pointing/Kinematics/Subsystem/Subsystem4/Subsystem12/Subsystem5 ==
  psi : Inport
  Constant1 : Constant  Value=[0 0 0; 0 0 0; 0 0 1]
  Constant2 : Constant  Value=[0 1 0; -1 0 0; 0 0 0]
  Constant3 : Constant  Value=[1 0 0; 0 1 0; 0 0 0]
  Cos : Trigonometry  Operator=cos
  Product : Product
  Product1 : Product
  Sin : Trigonometry
  Sum : Sum  Inputs=|+++
  3 : Outport
  wires:
  Sum/1 -> 3/1  "A3psi"
  psi/1 -> Sin/1, Cos/1  "psi"
  Product1/1 -> Sum/3
  Constant3/1 -> Product1/2
  Sin/1 -> Product/1
  Constant2/1 -> Product/2
  Cos/1 -> Product1/1
  Product/1 -> Sum/2
  Constant1/1 -> Sum/1

== system Nadir_Pointing/Kinematics/Subsystem/Subsystem4/Subsystem12/Subsystem6 ==
  phi : Inport
  Constant1 : Constant  Value=[0 0 0; 0 0 0; 0 0 1]
  Constant2 : Constant  Value=[0 1 0; -1 0 0; 0 0 0]
  Constant3 : Constant  Value=[1 0 0; 0 1 0; 0 0 0]
  Cos : Trigonometry  Operator=cos
  Product : Product
  Product1 : Product
  Sin : Trigonometry
  Sum : Sum  Inputs=|+++
  3 : Outport
  wires:
  phi/1 -> Cos/1, Sin/1
  Constant1/1 -> Sum/1
  Sum/1 -> 3/1  "A3phi"
  Sin/1 -> Product/1
  Constant2/1 -> Product/2
  Product/1 -> Sum/2
  Cos/1 -> Product1/1
  Constant3/1 -> Product1/2
  Product1/1 -> Sum/3

== matlab function Nadir_Pointing/CMG/MATLAB Function ==
  data: B input; y output
function y = pseudoinverse(B)

y=pinv(B);

end

== matlab function Nadir_Pointing/CMG/Singularity Condition/Subsystem/MATLAB Function ==
  data: B input; y output
function y = pseudoinverse(B)

y=pinv(B);

end
